simulink model "simpleMovement"  (R2017a)
settings: Solver=FixedStepDiscrete  StartTime=0.0  StopTime=Inf  FixedStep=0.1  RelTol=1e-3  EnableMultiTasking=on
model workspace (MAT data in the model file):
  SL_ROS_VariableLengthArrays_MaxSizes.CommonInfo.ArrayTruncateAction = 'EmitWarning'
  SL_ROS_VariableLengthArrays_MaxSizes.MsgTypeMap = containers.Map
  SL_ROS_VariableLengthArrays_MaxSizes.MsgTypeMap.serialization.keys = {'sensor_msgs/Image', 'sensor_msgs/LaserScan'}
  SL_ROS_VariableLengthArrays_MaxSizes.MsgTypeMap.serialization.values{1}(1).PropertyName = 'Data'
  SL_ROS_VariableLengthArrays_MaxSizes.MsgTypeMap.serialization.values{1}(1).DataType = 'uint8'
  SL_ROS_VariableLengthArrays_MaxSizes.MsgTypeMap.serialization.values{1}(1).MaxLength = 691200
  SL_ROS_VariableLengthArrays_MaxSizes.MsgTypeMap.serialization.values{1}(2).PropertyName = 'Encoding'
  SL_ROS_VariableLengthArrays_MaxSizes.MsgTypeMap.serialization.values{1}(2).DataType = 'uint8'
  SL_ROS_VariableLengthArrays_MaxSizes.MsgTypeMap.serialization.values{1}(2).MaxLength = 128
  SL_ROS_VariableLengthArrays_MaxSizes.MsgTypeMap.serialization.values{2}(1).PropertyName = 'Intensities'
  SL_ROS_VariableLengthArrays_MaxSizes.MsgTypeMap.serialization.values{2}(1).DataType = 'single'
  SL_ROS_VariableLengthArrays_MaxSizes.MsgTypeMap.serialization.values{2}(1).MaxLength = 1080
  SL_ROS_VariableLengthArrays_MaxSizes.MsgTypeMap.serialization.values{2}(2).PropertyName = 'Ranges'
  SL_ROS_VariableLengthArrays_MaxSizes.MsgTypeMap.serialization.values{2}(2).DataType = 'single'
  SL_ROS_VariableLengthArrays_MaxSizes.MsgTypeMap.serialization.values{2}(2).MaxLength = 1080
  SL_ROS_VariableLengthArrays_MaxSizes.MsgTypeMap.serialization.uniformity = 0
  SL_ROS_VariableLengthArrays_MaxSizes.MsgTypeMap.serialization.keyType = 'char'
  SL_ROS_VariableLengthArrays_MaxSizes.MsgTypeMap.serialization.valueType = 'any'
undefined symbols (not defined in the file): Angular, gray, Linear, sigbuilder_block
libraries: robotlib x6, aerolibanimutils x1, simulink x1
settings Model: Creator=The MathWorks, Inc.  LastModifiedBy=jcassett
settings DataIOCC: LimitDataPoints=on  SaveFormat=Array
settings OptimizationCC: LifeSpan=Inf  MaxStackSize=64
settings DebuggingCC: SolverPrmCheckMsg=warning  SFUnexpectedBacktrackingDiag=warning  SFNoUnconditionalDefaultTransitionDiag=warning  SFExecutionAtInitializationDiag=none
settings HardwareCC: ProdBitPerPointer=32  ProdBitPerSizeT=32  ProdBitPerPtrDiffT=32  ProdLargestAtomicFloat=None  ProdIntDivRoundTo=Undefined  ProdEndianess=Unspecified  ProdWordSize=32  ProdHWDeviceType=Generic->Unspecified (assume 32-bit Generic)  UseEmbeddedCoderFeatures=off
settings ModelReferenceCC: PropagateSignalLabelsOutOfModel=off
settings RTWCC: SystemTargetFile=ert.tlc  HardwareBoard=Robot Operating System (ROS)  TLCOptions=-aInlineSetEventsForThisBaseRateFcn=TLC_FALSE -aSuppressMultiTaskScheduler=TLC_FALSE -aRateBasedStepFcn=0  TemplateMakefile=ert_default_tmf  Description=Embedded Coder  Toolchain=Catkin  TargetLang=C++
settings ERTTargetCC: MultiwordLength=2048  ERTCustomFileBanners=off  SupportContinuousTime=on  SupportNonInlinedSFcns=on  RemoveResetFunc=off  SupportVariableSizeSignals=on  ModelStepFunctionPrototypeControlCompliant=off  ConvertIfToSwitch=off  SuppressUnreachableDefaultCases=off
settings ConfigComp: CovMetricSettings=dw  CovHtmlReporting=on  CovSaveCumulativeToWorkspaceVar=on  CovSaveSingleToWorkspaceVar=on  CovExternalEMLEnable=off  CovSFcnEnable=off

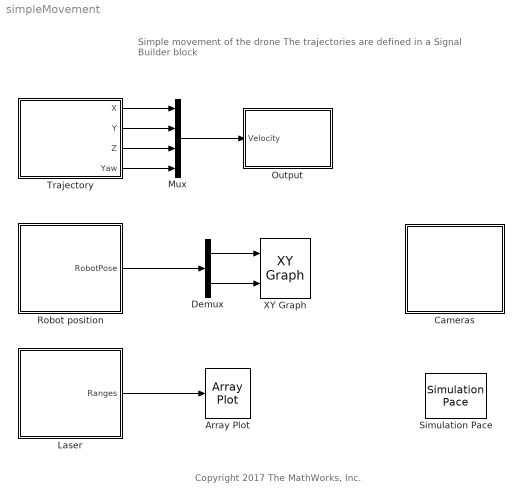
== system simpleMovement ==
  note: Simple movement of the drone
      | The trajectories are defined in a Signal Builder block
  note: Copyright 2017 The MathWorks, Inc.
  Array Plot : ArrayPlot
  Cameras : Subsystem
  Demux : Demux  Outputs=2
  Laser : Subsystem
  Mux : Mux
  Output : Subsystem
  Robot position : Subsystem
  Simulation Pace : aerolibanimutils/Simulation Pace  SimulationPace=1  SleepMode=MATLAB Thread  OutputPaceError=off  SampleTime=-1
  Trajectory : Subsystem  Tag=STV Subsys  LoadFcn=sigbuilder_block('load');  StartFcn=sigbuilder_block('start');  StopFcn=sigbuilder_block('stop');  ClipboardFcn=sigbuilder_block('clipboard');  mask(Sigbuilder block){tuvar=[0:10]}
      mask help: Simulink:masks:SigbuilderBlock_MD
      mask init:
      | if ~strcmp(get_param(bdroot(gcbh),'SimulationStatus'),'stopped') tuvar = sigbuilder_block('maskInit'); end
      settings: CopyFcn=sigbuilder_block('copy');  DeleteFcn=sigbuilder_block('delete');  ModelCloseFcn=sigbuilder_block('modelClose');  PreSaveFcn=sigbuilder_block('preSave');  PauseFcn=sigbuilder_block('pause');  ContinueFcn=sigbuilder_block('continue');  NameChangeFcn=sigbuilder_block('namechange');  OpenFcn=sigbuilder_block('open',[550.473 152.509 549.818 399.927 ]);  CloseFcn=sigbuilder_block('close');
      mask Display: plot(0, 0, 100, 100,[2, 2, 32, 32, 2], [68, 8, 8, 68, 68],[32, 2], [38, 38], [32, 19, 2],[53, 60, 44], [32, 17, 17, 2],[16, 16, 31, 31]);txt = getActiveGroup(gcbh);text(2, 100, txt,'verticalAlignment', 'top');
  XY Graph : simulink/Sinks/XY Graph  xmin=-10  xmax=30  ymin=-10  ymax=10  st=-1
  wires:
  Robot position/1(RobotPose) -> Demux/1
  Demux/1 -> XY Graph/1
  Demux/2 -> XY Graph/2
  Laser/1(Ranges) -> Array Plot/1
  Trajectory/1(X) -> Mux/1
  Trajectory/3(Z) -> Mux/3
  Mux/1 -> Output/1(Velocity)
  Trajectory/4(Yaw) -> Mux/4
  Trajectory/2(Y) -> Mux/2

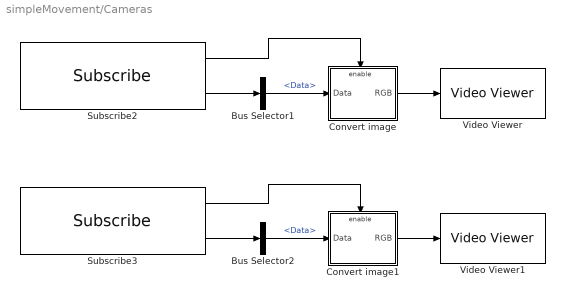
== system simpleMovement/Cameras ==
  Bus Selector1 : BusSelector  DialogController=Simulink.DDGSource_BusSelector  OutputSignals=Data
  Bus Selector2 : BusSelector  DialogController=Simulink.DDGSource_BusSelector  OutputSignals=Data
  Convert image : Subsystem
  Convert image1 : Subsystem
  Subscribe2 : robotlib/Subscribe  SourceLibraryInfo=This block requires Robotics System Toolbox  topicSource=Select from ROS network  topic=/quadrotor_1/front/image_raw  messageType=sensor_msgs/Image  sampleTime=-1  messageQueueLength=51
      settings: SourceProductBaseCode=RO
  Subscribe3 : robotlib/Subscribe  SourceLibraryInfo=This block requires Robotics System Toolbox  topicSource=Select from ROS network  topic=/quadrotor_1/bottom/image_raw  messageType=sensor_msgs/Image  sampleTime=-1  messageQueueLength=51
      settings: SourceProductBaseCode=RO
  Video Viewer : VideoViewer  colormapValue=gray(256)  FigPos=[1022.09090909091 508.545454545455 609.163636363637 376.145454545455]
  Video Viewer1 : VideoViewer  colormapValue=gray(256)  FigPos=[1013.36363636364 1003.38181818182 609.163636363636 376.145454545455]
  wires:
  Subscribe2/1 -> Convert image/Enable
  Convert image1/1(RGB) -> Video Viewer1/1
  Subscribe3/2 -> Bus Selector2/1
  Subscribe2/2 -> Bus Selector1/1
  Bus Selector1/1 -> Convert image/1(Data)  "<Data>"
  Bus Selector2/1 -> Convert image1/1(Data)  "<Data>"
  Subscribe3/1 -> Convert image1/Enable
  Convert image/1(RGB) -> Video Viewer/1

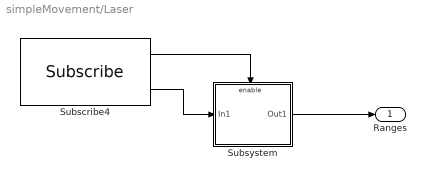
== system simpleMovement/Laser ==
  Subscribe4 : robotlib/Subscribe  SourceLibraryInfo=This block requires Robotics System Toolbox  topicSource=Select from ROS network  topic=/quadrotor_1/scan  messageType=sensor_msgs/LaserScan  sampleTime=-1  messageQueueLength=51
      settings: SourceProductBaseCode=RO
  Subsystem : Subsystem
  Ranges : Outport
  wires:
  Subsystem/1(Out1) -> Ranges/1
  Subscribe4/2 -> Subsystem/1(In1)
  Subscribe4/1 -> Subsystem/Enable

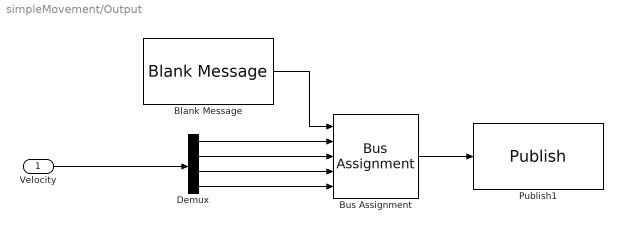
== system simpleMovement/Output ==
  Velocity : Inport
  Blank Message : robotlib/Blank Message  SourceLibraryInfo=This block requires Robotics System Toolbox  messageType=geometry_msgs/Twist  SampleTime=0
      settings: SourceProductBaseCode=RO
  Bus Assignment : BusAssignment  DialogController=Simulink.DDGSource_BusAssignment  AssignedSignals=Linear.X,Linear.Y,Linear.Z,Angular.Z
  Demux : Demux
  Publish1 : robotlib/Publish  SourceLibraryInfo=This block requires Robotics System Toolbox  topicSource=Select from ROS network  topic=/quadrotor_1/cmd_vel  messageType=geometry_msgs/Twist  messageQueueLength=105
      settings: SourceProductBaseCode=RO
  wires:
  Demux/2 -> Bus Assignment/3
  Demux/1 -> Bus Assignment/2
  Demux/3 -> Bus Assignment/4
  Demux/4 -> Bus Assignment/5
  Velocity/1 -> Demux/1
  Bus Assignment/1 -> Publish1/1
  Blank Message/1 -> Bus Assignment/1

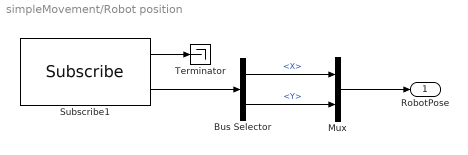
== system simpleMovement/Robot position ==
  Bus Selector : BusSelector  DialogController=Simulink.DDGSource_BusSelector  OutputSignals=Pose.Pose.Position.X,Pose.Pose.Position.Y
  Mux : Mux  Inputs=2
  Subscribe1 : robotlib/Subscribe  SourceLibraryInfo=This block requires Robotics System Toolbox  topicSource=Select from ROS network  topic=/quadrotor_1/ground_truth/state  messageType=nav_msgs/Odometry  sampleTime=-1  messageQueueLength=51
      settings: SourceProductBaseCode=RO
  Terminator : Terminator
  RobotPose : Outport
  wires:
  Subscribe1/2 -> Bus Selector/1
  Subscribe1/1 -> Terminator/1
  Bus Selector/1 -> Mux/1  "<X>"
  Bus Selector/2 -> Mux/2  "<Y>"
  Mux/1 -> RobotPose/1

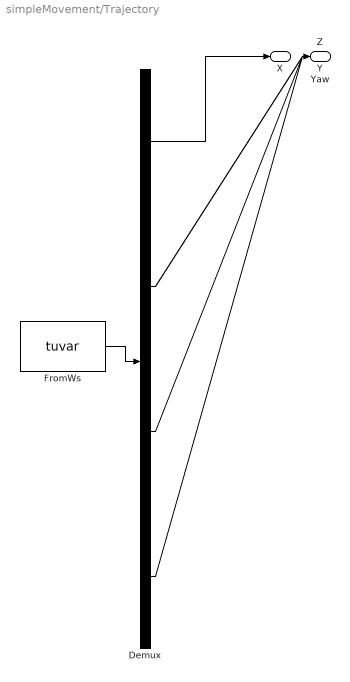
== system simpleMovement/Trajectory ==
  Demux : Demux  Tag=STV Demux
  FromWs : FromWorkspace  Tag=STV FromWs  VariableName=tuvar  SampleTime=0
      SigBuilderData=|
      | common.afterFinalStr = 'Extrapolate'
      | common.sampleTime = 0
      | dataSet(1).timeRange = [0 100]
      | dataSet(1).name = 'Steady'
      | dataSet(2).timeRange = [0 100]
      | dataSet(2).name = 'Up, Forward'
      | dataSet(3).timeRange = [0 100]
      | dataSet(3).name = 'Forward, Left'
      | sbobj.Groups(1).Name = 'Steady'
      | sbobj.Groups(1).Signals(1).Name = 'X'
      | sbobj.Groups(1).Signals(1).XData = [0 100]
      | sbobj.Groups(1).Signals(1).YData = [0 0]
      | sbobj.Groups(1).Signals(2).Name = 'Y'
      | sbobj.Groups(1).Signals(2).XData = [0 100]
      | sbobj.Groups(1).Signals(2).YData = [0 0]
      | sbobj.Groups(1).Signals(3).Name = 'Z'
      | sbobj.Groups(1).Signals(3).XData = [0 100]
      | sbobj.Groups(1).Signals(3).YData = [0 0]
      | sbobj.Groups(1).Signals(4).Name = 'Yaw'
      | sbobj.Groups(1).Signals(4).XData = [0 100]
      | sbobj.Groups(1).Signals(4).YData = [0 0]
      | sbobj.Groups(1).TimeRange = [0 100]
      | sbobj.Groups(2).Name = 'Up, Forward'
      | sbobj.Groups(2).Signals(1).Name = 'X'
      | sbobj.Groups(2).Signals(1).XData = [0 5 5 30 30 100]
      | sbobj.Groups(2).Signals(1).YData = [0 0 1 1 0 0]
      | sbobj.Groups(2).Signals(2).Name = 'Y'
      | sbobj.Groups(2).Signals(2).XData = [0 100]
      | sbobj.Groups(2).Signals(2).YData = [0 0]
      | sbobj.Groups(2).Signals(3).Name = 'Z'
      | sbobj.Groups(2).Signals(3).XData = [0 2 2 5 5 100]
      | sbobj.Groups(2).Signals(3).YData = [0 0 2 2 0 0]
      | sbobj.Groups(2).Signals(4).Name = 'Yaw'
      | sbobj.Groups(2).Signals(4).XData = [0 100]
      | sbobj.Groups(2).Signals(4).YData = [0 0]
      | sbobj.Groups(2).TimeRange = [0 100]
      | sbobj.Groups(3).Name = 'Forward, Left'
      | sbobj.Groups(3).Signals(1).Name = 'X'
      | sbobj.Groups(3).Signals(1).XData = [0 5 5 70 70 100]
      | sbobj.Groups(3).Signals(1).YData = [0 0 0.5 0.5 0 0]
      | sbobj.Groups(3).Signals(2).Name = 'Y'
      | sbobj.Groups(3).Signals(2).XData = [0 40 40 60 60 100]
      | sbobj.Groups(3).Signals(2).YData = [0 0 0.1 0.1 0 0]
      | sbobj.Groups(3).Signals(3).Name = 'Z'
      | sbobj.Groups(3).Signals(3).XData = [0 2 2 4 4 100]
      | sbobj.Groups(3).Signals(3).YData = [0 0 0.1 0.1 0 0]
      | sbobj.Groups(3).Signals(4).Name = 'Yaw'
      | sbobj.Groups(3).Signals(4).XData = [0 100]
      | sbobj.Groups(3).Signals(4).YData = [0 0]
      | sbobj.Groups(3).TimeRange = [0 100]
  X : Outport  Tag=STV Outport
  Y : Outport  Tag=STV Outport  Port=2
  Z : Outport  Tag=STV Outport  Port=3
  Yaw : Outport  Tag=STV Outport  Port=4
  wires:
  Demux/1 -> X/1
  FromWs/1 -> Demux/1
  Demux/2 -> Y/1
  Demux/3 -> Z/1
  Demux/4 -> Yaw/1

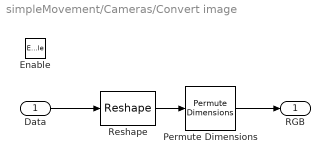
== system simpleMovement/Cameras/Convert image ==
  Data : Inport
  Enable : EnablePort
  Permute Dimensions : PermuteDimensions  Order=[3 2 1]
  Reshape : Reshape  OutputDimensionality=Customize  OutputDimensions=[3 640 360]
  RGB : Outport
  wires:
  Permute Dimensions/1 -> RGB/1
  Reshape/1 -> Permute Dimensions/1
  Data/1 -> Reshape/1

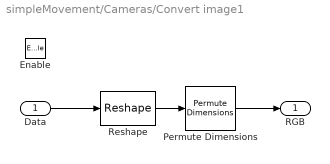
== system simpleMovement/Cameras/Convert image1 ==
  Data : Inport
  Enable : EnablePort
  Permute Dimensions : PermuteDimensions  Order=[3 2 1]
  Reshape : Reshape  OutputDimensionality=Customize  OutputDimensions=[3 640 360]
  RGB : Outport
  wires:
  Permute Dimensions/1 -> RGB/1
  Reshape/1 -> Permute Dimensions/1
  Data/1 -> Reshape/1

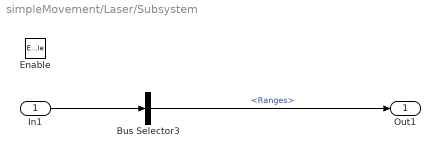
== system simpleMovement/Laser/Subsystem ==
  In1 : Inport
  Enable : EnablePort
  Bus Selector3 : BusSelector  DialogController=Simulink.DDGSource_BusSelector  OutputSignals=Ranges
  Out1 : Outport
  wires:
  Bus Selector3/1 -> Out1/1  "<Ranges>"
  In1/1 -> Bus Selector3/1
